simulink model "diodeclamped5lvl"  (R2023b)
settings: Solver=VariableStepAuto  StartTime=0.0  StopTime=0.3  RelTol=1e-3
libraries: spsIGBTDiodeLib x24, spsDiodeLib x18, simulink x12, spsSeriesRLCBranchLib x7, spsVoltageMeasurementLib x4, spsGroundLib x2, spsDCVoltageSourceLib x1, spsThreePhaseVIMeasurementLib x1, sps_lib x1
settings Model: Creator=user  LastModifiedBy=user

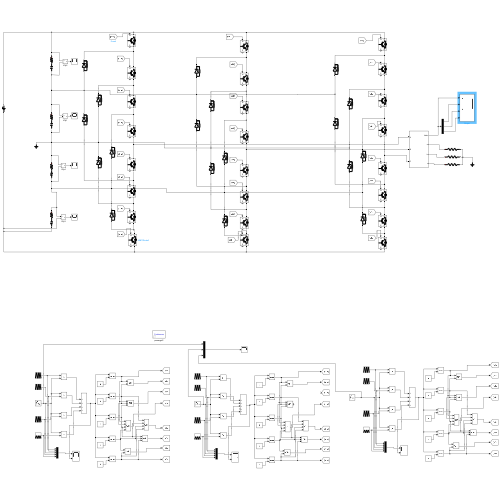
[thumbnail: Simulink's stored preview of the top-level diagram]
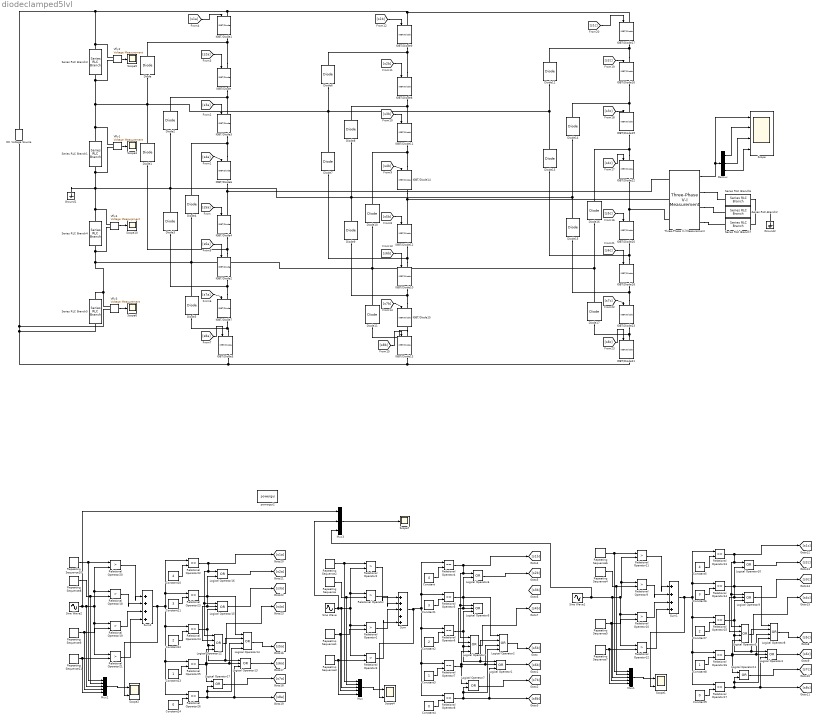
== system diodeclamped5lvl ==
  Constant : Constant  Value=4
  Constant1 : Constant  Value=3
  Constant10 : Constant  Value=4
  Constant11 : Constant  Value=3
  Constant12 : Constant  Value=2
  Constant13 : Constant
  Constant14 : Constant  Value=0
  Constant2 : Constant  Value=2
  Constant3 : Constant
  Constant4 : Constant  Value=0
  Constant5 : Constant  Value=4
  Constant6 : Constant  Value=3
  Constant7 : Constant  Value=2
  Constant8 : Constant
  Constant9 : Constant  Value=0
  DC Voltage Source : spsDCVoltageSourceLib/DC Voltage Source  Amplitude=100  Measurements=None
  Demux : Demux  Outputs=3
  Diode{,1..17} (18 alike) : spsDiodeLib/Diode  Ron=0.001  Lon=0  Vf=0.8  IC=0  UseSnubber=off  Rs=500  Cs=250e-9  Measurements=off
  Ground1 : spsGroundLib/Ground  LConnTagsString=a
  Ground2 : spsGroundLib/Ground  LConnTagsString=a
  IGBT/Diode{,1..23} (24 alike) : spsIGBTDiodeLib/IGBT//Diode  Ron=1e-3  Rs=1e5  Cs=inf  Measurements=on
  Logical Operator{,2..3,8,12,14} (6 alike) : Logic  Operator=OR  Inputs=4  AllPortsSameDT=off  OutDataTypeStr=boolean
  Logical Operator{1,4..5,9,13,15} (6 alike) : Logic  Operator=OR  Inputs=3  AllPortsSameDT=off  OutDataTypeStr=boolean
  Logical Operator{6..7,10..11,16..17} (6 alike) : Logic  Operator=OR  AllPortsSameDT=off  OutDataTypeStr=boolean
  Mux : Mux  Inputs=5
  Mux1 : Mux  Inputs=5
  Mux2 : Mux  Inputs=5
  Mux3 : Mux  Inputs=3
  Relational Operator{,1..3,9..12,18..21} (12 alike) : RelationalOperator  Operator=>  OutDataTypeStr=boolean  InputSameDT=off
  Relational Operator{4..8,13..17,22..26} (15 alike) : RelationalOperator  Operator===  OutDataTypeStr=boolean  InputSameDT=off
  Repeating Sequence : simulink/Sources/Repeating Sequence  rep_seq_t=[0 1 2 ]*[1/1000]  rep_seq_y=[0 1 0]
  Repeating Sequence1 : simulink/Sources/Repeating Sequence  rep_seq_t=[0 1 2]*[1/1000]  rep_seq_y=[-1 0 -1]
  Repeating Sequence10 : simulink/Sources/Repeating Sequence  rep_seq_t=[0 1 2 ]*[1/1000]  rep_seq_y=[1 2 1]
  Repeating Sequence11 : simulink/Sources/Repeating Sequence  rep_seq_t=[0 1 2]*[1/1000]  rep_seq_y=[-2 -1 -2]
  Repeating Sequence2 : simulink/Sources/Repeating Sequence  rep_seq_t=[0 1 2 ]*[1/1000]  rep_seq_y=[1 2 1]
  Repeating Sequence3 : simulink/Sources/Repeating Sequence  rep_seq_t=[0 1 2]*[1/1000]  rep_seq_y=[-2 -1 -2]
  Repeating Sequence4 : simulink/Sources/Repeating Sequence  rep_seq_t=[0 1 2 ]*[1/1000]  rep_seq_y=[0 1 0]
  Repeating Sequence5 : simulink/Sources/Repeating Sequence  rep_seq_t=[0 1 2]*[1/1000]  rep_seq_y=[-1 0 -1]
  Repeating Sequence6 : simulink/Sources/Repeating Sequence  rep_seq_t=[0 1 2 ]*[1/1000]  rep_seq_y=[1 2 1]
  Repeating Sequence7 : simulink/Sources/Repeating Sequence  rep_seq_t=[0 1 2]*[1/1000]  rep_seq_y=[-2 -1 -2]
  Repeating Sequence8 : simulink/Sources/Repeating Sequence  rep_seq_t=[0 1 2 ]*[1/1000]  rep_seq_y=[0 1 0]
  Repeating Sequence9 : simulink/Sources/Repeating Sequence  rep_seq_t=[0 1 2]*[1/1000]  rep_seq_y=[-1 0 -1]
  Scope : Scope  NumInputPorts=4
  Scope1 : Scope  NumInputPorts=2
  Scope{3,5..7,10} (5 alike) : Scope
  Scope2 : Scope  NumInputPorts=2
  Scope4 : Scope  NumInputPorts=2
  Series RLC Branch{1,3..5} (4 alike) : spsSeriesRLCBranchLib/Series RLC Branch  LConnTagsString=__new0  RConnTagsString=__new0  BranchType=RC  Resistance=0.01  Inductance=20e-6  SetiL0=off  InitialCurrent=0  Capacitance=4.7e-3  Setx0=off  InitialVoltage=0  Measurements=None
  Series RLC Branch2 : spsSeriesRLCBranchLib/Series RLC Branch  LConnTagsString=__new0  RConnTagsString=__new0  BranchType=R  Resistance=100  Inductance=20e-6  SetiL0=off  InitialCurrent=0  Capacitance=4.7e-3  Setx0=off  InitialVoltage=0  Measurements=None
  Series RLC Branch6 : spsSeriesRLCBranchLib/Series RLC Branch  LConnTagsString=__new0  RConnTagsString=__new0  BranchType=R  Resistance=500  Inductance=20e-6  SetiL0=off  InitialCurrent=0  Capacitance=4.7e-3  Setx0=off  InitialVoltage=0  Measurements=None
  Series RLC Branch7 : spsSeriesRLCBranchLib/Series RLC Branch  LConnTagsString=__new0  RConnTagsString=__new0  BranchType=R  Resistance=250  Inductance=20e-6  SetiL0=off  InitialCurrent=0  Capacitance=4.7e-3  Setx0=off  InitialVoltage=0  Measurements=None
  Sine Wave : Sin  Amplitude=2  Frequency=2*pi*50  Phase=4*pi/3  SampleTime=0
  Sine Wave1 : Sin  Amplitude=2  Frequency=2*pi*50  Phase=2*pi/3  SampleTime=0
  Sine Wave2 : Sin  Amplitude=2  Frequency=2*pi*50  SampleTime=0
  Sum : Sum  Inputs=|+++++
  Sum1 : Sum  Inputs=|++++
  Sum2 : Sum  Inputs=|++++
  Three-Phase V-I Measurement : spsThreePhaseVIMeasurementLib/Three-Phase V-I Measurement  VoltageMeasurement=phase-to-ground  SetLabelV=off  LabelV=Vabc  Vpu=off  VpuLL=off  CurrentMeasurement=no  SetLabelI=off  LabelI=Iabc  Ipu=off  Pbase=100e6  Vbase=500e3  OutputType=Complex  PhasorSimulation=off  PSBequivalent=0
  Vfly{1..4} (4 alike) : spsVoltageMeasurementLib/Voltage Measurement  PhasorSimulation=off  OutputType=Complex  PSBequivalent=0
  powergui2 : sps_lib/powergui  Priority=1  SimulationMode=Continuous  SampleTime=5e-4  frequency=60  Iterations=50  frequencyindice=0  Pbase=100e6  ErrMax=1e-4  UnitsV=kV  UnitsW=MW  buscounter=0  FunctionMessages=off  echomessages=off  EnableUseOfTLC=off  CurrentSourceSwitches=on  DisableSnubberDevices=off  DisableRonSwitches=off  DisableVfSwitches=off  DisplayEquations=off  AutomaticDiscreteSolvers=off  SolverType=Tustin/Backward Euler (TBE)  Interpol=off  ExternalGateDelay=off  methode=off  Ts=10  x0status=blocks  SPID=off  SwTol=0  HookPort=off  NonlinearTolerance=1e-4  nMaxIteration=100  ContinueOnMaxIteration=off  RestoreLinks=warning  ResistiveCurrentMeasurement=off  Frange=[0:2:500]  Ylog=off  Xlog=on  ShowGrid=off  save=off  variable=ZData  structure=ScopeData3  ZoomFFT=off  StartTime=0.0  cycles=1  DisplayStyle=1  fundamental=50  FreqAxis=off  MaxFrequency=1000  frequencyindicesteady=1  RmsSteady=1  display=off
  wires:
  Logical Operator2/1 -> [s5b]
  Relational Operator6/1 -> Logical Operator2/2, Logical Operator1/1, Logical Operator/3, Logical Operator5/3
  Logical Operator7/1 -> [s7b]
  Logical Operator/1 -> [s4b]
  Relational Operator4/1 -> Logical Operator6/1, Logical Operator/1, Logical Operator5/1, [s1b]
  Constant2/1 -> Relational Operator6/2
  Relational Operator1/1 -> Sum/3
  Relational Operator8/1 -> Logical Operator2/4, Logical Operator7/2, Logical Operator1/3, [s8b]
  Constant4/1 -> Relational Operator8/2
  Logical Operator6/1 -> [s2b]
  Relational Operator2/1 -> Sum/1
  Repeating Sequence3/1 -> Mux/5, Relational Operator3/2
  Sum/1 -> Relational Operator8/1, Relational Operator7/1, Relational Operator6/1, Relational Operator5/1, Relational Operator4/1, Scope4/2
  Constant3/1 -> Relational Operator7/2
  Constant1/1 -> Relational Operator5/2
  Relational Operator/1 -> Sum/2
  Repeating Sequence2/1 -> Mux/1, Relational Operator2/1
  Relational Operator3/1 -> Sum/5
  Repeating Sequence/1 -> Mux/2, Relational Operator/2
  Relational Operator5/1 -> Logical Operator2/1, Logical Operator6/2, Logical Operator5/2, Logical Operator/2
  Mux/1 -> Scope4/1
  Relational Operator7/1 -> Logical Operator7/1, Logical Operator2/3, Logical Operator1/2, Logical Operator/4
  Constant/1 -> Relational Operator4/2
  Sine Wave/1 -> Mux3/2, Mux/3, Relational Operator1/1, Relational Operator3/1, Relational Operator2/2, Relational Operator/1
  Repeating Sequence1/1 -> Mux/4, Relational Operator1/2
  Logical Operator1/1 -> [s6b]
  Logical Operator8/1 -> [s5c]
  Relational Operator15/1 -> Logical Operator8/2, Logical Operator4/1, Logical Operator3/3, Logical Operator9/3
  Logical Operator9/1 -> [s3c]
  Logical Operator11/1 -> [s7c]
  Logical Operator3/1 -> [s4c]
  Relational Operator13/1 -> Logical Operator10/1, Logical Operator3/1, Logical Operator9/1, [s1c]
  Constant7/1 -> Relational Operator15/2
  Relational Operator10/1 -> Sum1/3
  Relational Operator17/1 -> Logical Operator8/4, Logical Operator11/2, Logical Operator4/3, [s8c]
  Constant9/1 -> Relational Operator17/2
  Logical Operator10/1 -> [s2c]
  Relational Operator11/1 -> Sum1/1
  Repeating Sequence7/1 -> Mux1/5, Relational Operator12/2
  Sum1/1 -> Scope1/2, Relational Operator17/1, Relational Operator16/1, Relational Operator15/1, Relational Operator14/1, Relational Operator13/1
  Constant8/1 -> Relational Operator16/2
  Constant6/1 -> Relational Operator14/2
  Relational Operator9/1 -> Sum1/2
  Repeating Sequence6/1 -> Mux1/1, Relational Operator11/1
  Relational Operator12/1 -> Sum1/4
  Repeating Sequence4/1 -> Mux1/2, Relational Operator9/2
  Relational Operator14/1 -> Logical Operator8/1, Logical Operator10/2, Logical Operator9/2, Logical Operator3/2
  Mux1/1 -> Scope1/1
  Relational Operator16/1 -> Logical Operator11/1, Logical Operator8/3, Logical Operator4/2, Logical Operator3/4
  Constant5/1 -> Relational Operator13/2
  Sine Wave1/1 -> Mux1/3, Relational Operator10/1, Relational Operator12/1, Relational Operator11/2, Relational Operator9/1, Mux3/3
  Repeating Sequence5/1 -> Mux1/4, Relational Operator10/2
  Logical Operator4/1 -> [s6c]
  Logical Operator14/1 -> [s5a]
  Relational Operator24/1 -> Logical Operator14/2, Logical Operator13/1, Logical Operator12/3, Logical Operator15/3
  Logical Operator15/1 -> [s3a]
  Logical Operator17/1 -> [s7a]
  Logical Operator12/1 -> [s4a]
  Relational Operator22/1 -> Logical Operator16/1, Logical Operator12/1, Logical Operator15/1, [s1a]
  Constant12/1 -> Relational Operator24/2
  Relational Operator19/1 -> Sum2/3
  Relational Operator26/1 -> Logical Operator14/4, Logical Operator17/2, Logical Operator13/3, [s8a]
  Constant14/1 -> Relational Operator26/2
  Logical Operator16/1 -> [s2a]
  Relational Operator20/1 -> Sum2/1
  Repeating Sequence11/1 -> Mux2/5, Relational Operator21/2
  Sum2/1 -> Scope2/2, Relational Operator26/1, Relational Operator25/1, Relational Operator24/1, Relational Operator23/1, Relational Operator22/1
  Constant13/1 -> Relational Operator25/2
  Constant11/1 -> Relational Operator23/2
  Relational Operator18/1 -> Sum2/2
  Repeating Sequence10/1 -> Mux2/1, Relational Operator20/1
  Relational Operator21/1 -> Sum2/4
  Repeating Sequence8/1 -> Mux2/2, Relational Operator18/2
  Relational Operator23/1 -> Logical Operator14/1, Logical Operator16/2, Logical Operator15/2, Logical Operator12/2
  Mux2/1 -> Scope2/1
  Relational Operator25/1 -> Logical Operator17/1, Logical Operator14/3, Logical Operator13/2, Logical Operator12/4
  Constant10/1 -> Relational Operator22/2
  Sine Wave2/1 -> Relational Operator20/2, Relational Operator18/1, Relational Operator19/1, Relational Operator21/1, Mux2/3, Mux3/1
  Repeating Sequence9/1 -> Mux2/4, Relational Operator19/2
  Logical Operator13/1 -> [s6a]
  [s4a] -> IGBT/Diode6/1
  Vfly4/1 -> Scope10/1
  Vfly3/1 -> Scope6/1
  [s7a] -> IGBT/Diode7/1
  [s6a] -> IGBT/Diode2/1
  [s2a] -> IGBT/Diode/1
  [s5a] -> IGBT/Diode4/1
  [s3a] -> IGBT/Diode3/1
  Vfly1/1 -> Scope3/1
  Vfly2/1 -> Scope5/1
  [s8a] -> IGBT/Diode5/1
  [s1a] -> IGBT/Diode1/1
  [s3b] -> IGBT/Diode11/1
  [s8b] -> IGBT/Diode13/1
  [s1b] -> IGBT/Diode9/1
  [s2b] -> IGBT/Diode8/1
  [s4b] -> IGBT/Diode14/1
  [s7b] -> IGBT/Diode15/1
  [s5b] -> IGBT/Diode12/1
  [s6b] -> IGBT/Diode10/1
  [s3c] -> IGBT/Diode19/1
  [s8c] -> IGBT/Diode21/1
  [s1c] -> IGBT/Diode17/1
  [s2c] -> IGBT/Diode16/1
  [s4c] -> IGBT/Diode22/1
  [s7c] -> IGBT/Diode23/1
  [s5c] -> IGBT/Diode20/1
  [s6c] -> IGBT/Diode18/1
  Three-Phase V-I Measurement/1 -> Scope/1, Demux/1
  Demux/1 -> Scope/2
  Demux/2 -> Scope/3
  Demux/3 -> Scope/4
  Mux3/1 -> Scope7/1
  connections:
  Series RLC Branch5/RConn1 -- IGBT/Diode21/RConn1 -- IGBT/Diode13/RConn1 -- IGBT/Diode5/RConn1 -- DC Voltage Source/LConn1 -- Vfly3/LConn2
  IGBT/Diode6/LConn1 -- IGBT/Diode3/RConn1 -- Diode4/RConn1
  Diode17/RConn1 -- Diode11/RConn1 -- Diode4/LConn1 -- Diode5/RConn1 -- Series RLC Branch4/RConn1 -- Vfly4/LConn2 -- Vfly3/LConn1 -- Series RLC Branch5/LConn1 -- Diode10/LConn1 -- Diode16/LConn1
  IGBT/Diode6/RConn1 -- Three-Phase V-I Measurement/LConn1 -- IGBT/Diode4/LConn1
  IGBT/Diode5/LConn1 -- IGBT/Diode7/RConn1 -- Diode5/LConn1
  Diode2/RConn1 -- IGBT/Diode/RConn1 -- IGBT/Diode3/LConn1
  Series RLC Branch3/LConn1 -- Vfly2/LConn1 -- IGBT/Diode17/LConn1 -- IGBT/Diode9/LConn1 -- IGBT/Diode1/LConn1 -- DC Voltage Source/RConn1
  Diode13/RConn1 -- Diode6/LConn1 -- Diode7/RConn1 -- Diode/LConn1 -- Diode1/RConn1 -- Series RLC Branch1/LConn1 -- Vfly1/LConn1 -- Vfly2/LConn2 -- Series RLC Branch3/RConn1 -- Diode12/LConn1
  IGBT/Diode/LConn1 -- IGBT/Diode1/RConn1 -- Diode/RConn1
  Diode15/RConn1 -- Diode14/LConn1 -- Ground1/LConn1 -- Vfly4/LConn1 -- Series RLC Branch4/LConn1 -- Vfly1/LConn2 -- Series RLC Branch1/RConn1 -- Diode2/LConn1 -- Diode3/RConn1 -- Diode8/LConn1 -- Diode9/RConn1
  IGBT/Diode2/LConn1 -- IGBT/Diode4/RConn1 -- Diode1/LConn1
  IGBT/Diode7/LConn1 -- IGBT/Diode2/RConn1 -- Diode3/LConn1
  IGBT/Diode8/LConn1 -- IGBT/Diode9/RConn1 -- Diode6/RConn1
  IGBT/Diode13/LConn1 -- IGBT/Diode15/RConn1 -- Diode11/LConn1
  Diode8/RConn1 -- IGBT/Diode8/RConn1 -- IGBT/Diode11/LConn1
  IGBT/Diode15/LConn1 -- IGBT/Diode10/RConn1 -- Diode9/LConn1
  IGBT/Diode14/RConn1 -- IGBT/Diode12/LConn1 -- Three-Phase V-I Measurement/LConn2
  IGBT/Diode14/LConn1 -- IGBT/Diode11/RConn1 -- Diode10/RConn1
  IGBT/Diode10/LConn1 -- IGBT/Diode12/RConn1 -- Diode7/LConn1
  IGBT/Diode16/LConn1 -- IGBT/Diode17/RConn1 -- Diode12/RConn1
  IGBT/Diode21/LConn1 -- IGBT/Diode23/RConn1 -- Diode17/LConn1
  Diode14/RConn1 -- IGBT/Diode16/RConn1 -- IGBT/Diode19/LConn1
  IGBT/Diode23/LConn1 -- IGBT/Diode18/RConn1 -- Diode15/LConn1
  IGBT/Diode22/RConn1 -- IGBT/Diode20/LConn1 -- Three-Phase V-I Measurement/LConn3
  IGBT/Diode22/LConn1 -- IGBT/Diode19/RConn1 -- Diode16/RConn1
  IGBT/Diode18/LConn1 -- IGBT/Diode20/RConn1 -- Diode13/LConn1
  Three-Phase V-I Measurement/RConn1 -- Series RLC Branch6/LConn1
  Three-Phase V-I Measurement/RConn2 -- Series RLC Branch2/LConn1
  Three-Phase V-I Measurement/RConn3 -- Series RLC Branch7/LConn1
  Series RLC Branch6/RConn1 -- Ground2/LConn1 -- Series RLC Branch7/RConn1 -- Series RLC Branch2/RConn1
